simulink model "RLC_done2"  (R2020a)
settings: Solver=VariableStepAuto  StartTime=0.0  StopTime=50  RelTol=1e-3
settings Model: Creator=Dell  LastModifiedBy=Dell

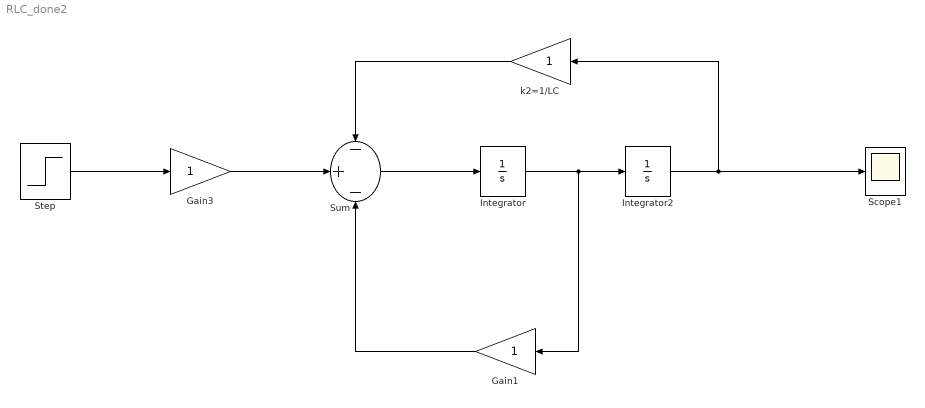
== system RLC_done2 ==
  Gain1 : Gain
  Gain3 : Gain
  Integrator : Integrator
  Integrator2 : Integrator
  Scope1 : Scope
  Step : Step  SampleTime=0
  Sum : Sum  Inputs=-+-
  k2=1/LC : Gain
  wires:
  k2=1/LC/1 -> Sum/1
  Sum/1 -> Integrator/1
  Step/1 -> Gain3/1
  Gain3/1 -> Sum/2
  Integrator/1 -> Gain1/1, Integrator2/1
  Gain1/1 -> Sum/3
  Integrator2/1 -> k2=1/LC/1, Scope1/1
